simulink model "inputs"  (R2022b)
settings: Solver=VariableStepAuto  StartTime=0.0  StopTime=50  RelTol=1e-3
undefined symbols (not defined in the file or in its folder): sigbuilder_block
libraries: dspsrcs4 x1

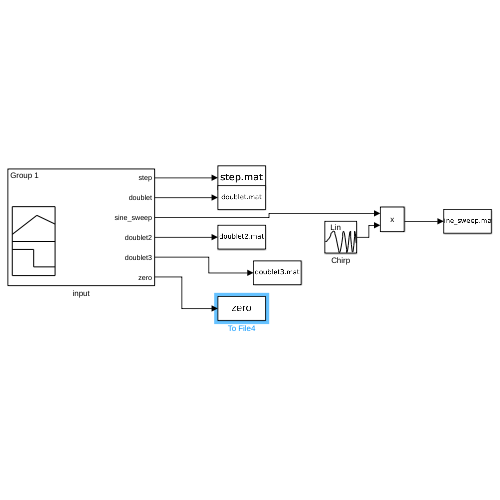
[thumbnail: Simulink's stored preview of the top-level diagram]
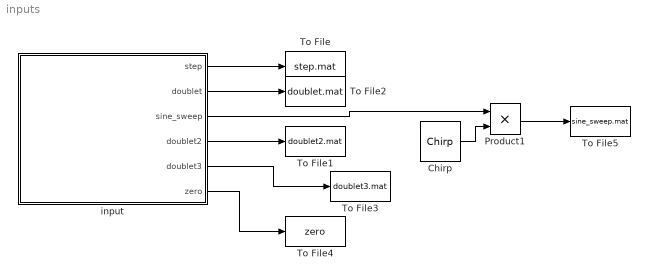
== system inputs ==
  Chirp : dspsrcs4/Chirp  sweep=Linear  mode=Unidirectional  f0=0  f1=3  t1=20  Tsweep=20  phase=0  Ts=0.02  spf=1  datatype=Double  OutputFrames=off
  Product1 : Product
  To File : ToFile  Filename=step.mat  MatrixName=step  SaveFormat=Timeseries  SampleTime=0.02
  To File1 : ToFile  Filename=doublet2.mat  MatrixName=doublet2  SaveFormat=Timeseries  SampleTime=0.02
  To File2 : ToFile  Filename=doublet.mat  MatrixName=doublet  SaveFormat=Timeseries  SampleTime=0.02
  To File3 : ToFile  Filename=doublet3.mat  MatrixName=doublet3  SaveFormat=Timeseries  SampleTime=0.02
  To File4 : ToFile  Filename=zero  MatrixName=zero  SaveFormat=Timeseries  SampleTime=0.02
  To File5 : ToFile  Filename=sine_sweep.mat  MatrixName=sine_sweep  SaveFormat=Timeseries  SampleTime=0.02
  input : Subsystem  Tag=STV Subsys  LoadFcn=sigbuilder_block('load',[175.5 193.5 1109.25 571.5 ]);  StartFcn=sigbuilder_block('start');  StopFcn=sigbuilder_block('stop');  ClipboardFcn=sigbuilder_block('clipboard');  mask(Sigbuilder block){tuvar=[0:10]}
      mask help: Simulink:masks:SigbuilderBlock_MD
      mask init:
      | if ~strcmp(get_param(bdroot(gcbh),'SimulationStatus'),'stopped') tuvar = sigbuilder_block('maskInit'); end
  wires:
  input/1(step) -> To File/1
  input/2(doublet) -> To File2/1
  input/3(sine_sweep) -> Product1/1
  Chirp/1 -> Product1/2
  Product1/1 -> To File5/1
  input/4(doublet2) -> To File1/1
  input/5(doublet3) -> To File3/1
  input/6(zero) -> To File4/1

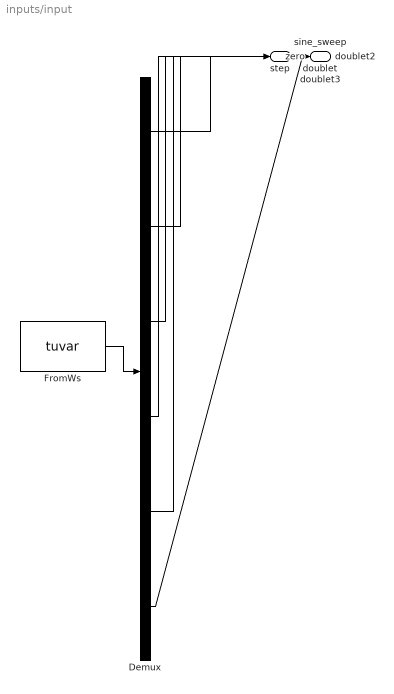
== system inputs/input ==
  Demux : Demux  Tag=STV Demux  Outputs=6
  FromWs : FromWorkspace  Tag=STV FromWs  VariableName=tuvar  SampleTime=1/50
      SigBuilderData=|
      | common.afterFinalStr = 'Extrapolate'
      | common.sampleTime = '1/50'
      | dataSet.timeRange = [0 30]
      | dataSet.name = 'Group 1'
      | sbobj.Groups.Name = 'Group 1'
      | sbobj.Groups.Signals(1).Name = 'step'
      | sbobj.Groups.Signals(1).XData = [0 1.98 1.98 5.02 30]
      | sbobj.Groups.Signals(1).YData = [0 0 0.1 0.1 0.1]
      | sbobj.Groups.Signals(2).Name = 'doublet'
      | sbobj.Groups.Signals(2).XData = [0 1.1 1.1 1.6 1.6 2.02 2.02 30]
      | sbobj.Groups.Signals(2).YData = [0 0 0.1 0.1 -0.1 -0.1 0 0]
      | sbobj.Groups.Signals(3).Name = 'sine_sweep'
      | sbobj.Groups.Signals(3).XData = [0 1.98 1.98 30]
      | sbobj.Groups.Signals(3).YData = [0 0 0.1 0.1]
      | sbobj.Groups.Signals(4).Name = 'doublet2'
      | sbobj.Groups.Signals(4).XData = [0 7.35 7.35 7.8 7.8 8.2 8.2 30]
      | sbobj.Groups.Signals(4).YData = [0 0 0.1 0.1 -0.1 -0.1 0 0]
      | sbobj.Groups.Signals(5).Name = 'doublet3'
      | sbobj.Groups.Signals(5).XData = [0 22.7 22.7 23.15 23.15 23.6 23.6 30]
      | sbobj.Groups.Signals(5).YData = [0 0 0.1 0.1 -0.1 -0.1 0 0]
      | sbobj.Groups.Signals(6).Name = 'zero'
      | sbobj.Groups.Signals(6).XData = [0 12 18 30]
      | sbobj.Groups.Signals(6).YData = [0 0 0 0]
      | sbobj.Groups.TimeRange = [0 30]
  step : Outport  Tag=STV Outport
  doublet : Outport  Tag=STV Outport  Port=2
  sine_sweep : Outport  Tag=STV Outport  Port=3
  doublet2 : Outport  Tag=STV Outport  Port=4
  doublet3 : Outport  Tag=STV Outport  Port=5
  zero : Outport  Tag=STV Outport  Port=6
  wires:
  Demux/1 -> step/1
  FromWs/1 -> Demux/1
  Demux/2 -> doublet/1
  Demux/3 -> sine_sweep/1
  Demux/4 -> doublet2/1
  Demux/5 -> doublet3/1
  Demux/6 -> zero/1
